simulink model "nnROSNode"  (R2019a)
settings: Solver=FixedStepAuto  StartTime=0.0  StopTime=inf  FixedStep=0.1667  RelTol=1e-3
model workspace (MAT data in the model file):
  SL_ROS_VariableLengthArrays_MaxSizes.CommonInfo.ArrayTruncateAction = 'EmitWarning'
  SL_ROS_VariableLengthArrays_MaxSizes.MsgTypeMap = containers.Map
  SL_ROS_VariableLengthArrays_MaxSizes.MsgTypeMap.serialization.keys = {'dronecomms/droneOut32', 'dronecomms/pidIn32', 'rospy_tutorials/Floats', 'std_msgs/Float32MultiArray'}
  SL_ROS_VariableLengthArrays_MaxSizes.MsgTypeMap.serialization.values{1}.PropertyName = 'Data'
  SL_ROS_VariableLengthArrays_MaxSizes.MsgTypeMap.serialization.values{1}.DataType = 'single'
  SL_ROS_VariableLengthArrays_MaxSizes.MsgTypeMap.serialization.values{1}.MaxLength = 20
  SL_ROS_VariableLengthArrays_MaxSizes.MsgTypeMap.serialization.values{2}.PropertyName = 'Data'
  SL_ROS_VariableLengthArrays_MaxSizes.MsgTypeMap.serialization.values{2}.DataType = 'single'
  SL_ROS_VariableLengthArrays_MaxSizes.MsgTypeMap.serialization.values{2}.MaxLength = 16
  SL_ROS_VariableLengthArrays_MaxSizes.MsgTypeMap.serialization.values{3}.PropertyName = 'Data'
  SL_ROS_VariableLengthArrays_MaxSizes.MsgTypeMap.serialization.values{3}.DataType = 'single'
  SL_ROS_VariableLengthArrays_MaxSizes.MsgTypeMap.serialization.values{3}.MaxLength = 20
  SL_ROS_VariableLengthArrays_MaxSizes.MsgTypeMap.serialization.values{4}.PropertyName = 'Data'
  SL_ROS_VariableLengthArrays_MaxSizes.MsgTypeMap.serialization.values{4}.DataType = 'single'
  SL_ROS_VariableLengthArrays_MaxSizes.MsgTypeMap.serialization.values{4}.MaxLength = 16
  SL_ROS_VariableLengthArrays_MaxSizes.MsgTypeMap.serialization.uniformity = 0
  SL_ROS_VariableLengthArrays_MaxSizes.MsgTypeMap.serialization.keyType = 'char'
  SL_ROS_VariableLengthArrays_MaxSizes.MsgTypeMap.serialization.valueType = 'any'
values from neighbouring files (symbols this model uses):
  maxDeviationTarget = [0.1 0.1 0.1]    [oldNN.mat]
undefined symbols (not defined in the file or in its folder): Data, Data_SL_Info, g, rho, Vehicle
libraries: neural x70, robotlib x3, dspstat3 x2, dynamicsLibrary x1, sharedtransform x1
(part 1 of 2)

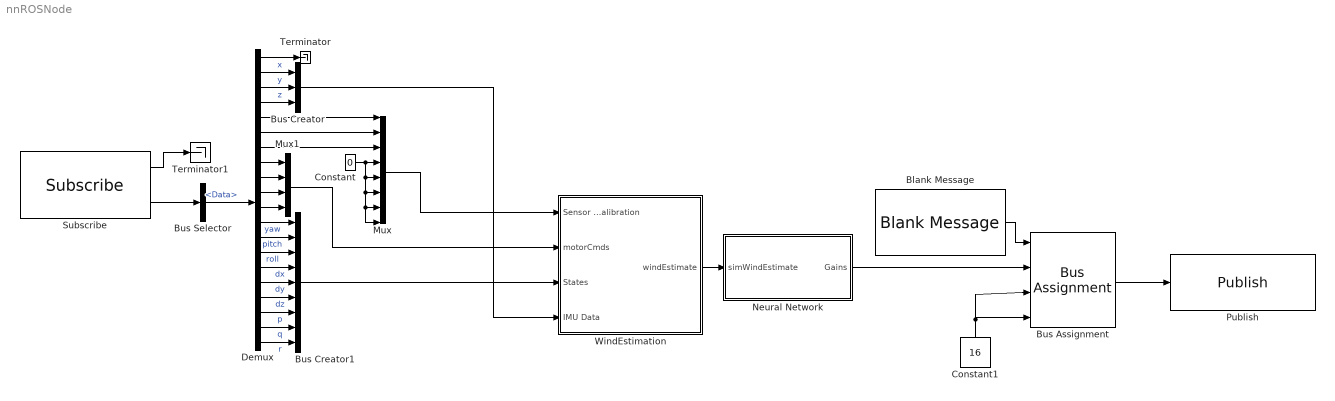
== system nnROSNode ==
  Blank Message : robotlib/Blank Message  messageClass=Message  entityType=dronecomms/pidIn32  messageType=dronecomms/pidIn32  SampleTime=inf
  Bus Assignment : BusAssignment  AssignedSignals=Data,Data_SL_Info.CurrentLength,Data_SL_Info.ReceivedLength
  Bus Creator : BusCreator  Inputs=3
  Bus Creator1 : BusCreator  Inputs=9
  Bus Selector : BusSelector  OutputSignals=Data
  Constant : Constant  Value=0  OutDataTypeStr=single
  Constant1 : Constant  Value=16  OutDataTypeStr=uint32
  Demux : Demux  Outputs=20
  Mux : Mux  Inputs=8
  Mux1 : Mux
  Neural Network : Subsystem
  Publish : robotlib/Publish  topicSource=Specify your own  topic=/pid_gains  messageType=dronecomms/pidIn32  messageQueueLength=1
  Subscribe : robotlib/Subscribe  topicSource=Select from ROS network  topic=/drone_data_recieved  messageType=dronecomms/droneOut32  sampleTime=-1  messageQueueLength=1
  Terminator : Terminator
  Terminator1 : Terminator
  WindEstimation : Subsystem
  wires:
  WindEstimation/1(windEstimate) -> Neural Network/1(simWindEstimate)
  Demux/2 -> Bus Creator/1  "x"
  Demux/3 -> Bus Creator/2  "y"
  Demux/4 -> Bus Creator/3  "z"
  Demux/1 -> Terminator/1
  Demux/8 -> Mux1/1
  Demux/9 -> Mux1/2
  Demux/10 -> Mux1/3
  Demux/11 -> Mux1/4
  Demux/12 -> Bus Creator1/1  "yaw"
  Demux/13 -> Bus Creator1/2  "pitch"
  Demux/14 -> Bus Creator1/3  "roll"
  Demux/15 -> Bus Creator1/4  "dx"
  Demux/16 -> Bus Creator1/5  "dy"
  Demux/17 -> Bus Creator1/6  "dz"
  Demux/18 -> Bus Creator1/7  "p"
  Demux/19 -> Bus Creator1/8  "q"
  Demux/20 -> Bus Creator1/9  "r"
  Demux/5 -> Mux/1
  Demux/6 -> Mux/2
  Demux/7 -> Mux/3
  Mux/1 -> WindEstimation/1(Sensor Calibration)
  Constant/1 -> Mux/8, Mux/7, Mux/6, Mux/5, Mux/4
  Mux1/1 -> WindEstimation/2(motorCmds)
  Bus Creator1/1 -> WindEstimation/3(States)
  Bus Creator/1 -> WindEstimation/4(IMU Data)
  Blank Message/1 -> Bus Assignment/1
  Bus Assignment/1 -> Publish/1
  Neural Network/1(Gains) -> Bus Assignment/2
  Subscribe/1 -> Terminator1/1
  Bus Selector/1 -> Demux/1  "<Data>"
  Constant1/1 -> Bus Assignment/4, Bus Assignment/3
  Subscribe/2 -> Bus Selector/1

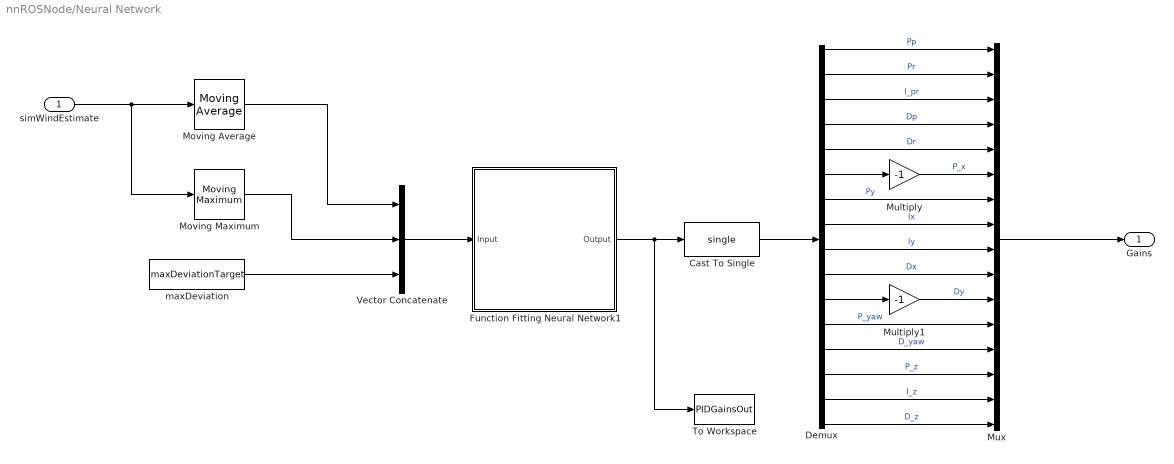
== system nnROSNode/Neural Network ==
  simWindEstimate : Inport
  Cast To Single : DataTypeConversion  OutDataTypeStr=single
  Demux : Demux  Outputs=16
  Function Fitting Neural Network1 : Subsystem
      mask help: Function Fitting Neural Network
  Moving Average : dspstat3/Moving Average  Method=Sliding window  ForgettingFactorPort=off  SpecifyWindowLength=on  WindowLength=100  ForgettingFactor=0.9  SimulateUsing=Code generation
  Moving Maximum : dspstat3/Moving Maximum  SpecifyWindowLength=on  WindowLength=100  SimulateUsing=Code generation
  Multiply : Gain  Gain=-1
  Multiply1 : Gain  Gain=-1
  Mux : Mux  Inputs=16
  To Workspace : ToWorkspace  VariableName=PIDGainsOut  SaveFormat=Structure With Time  SampleTime=-1
  Vector Concatenate : Concatenate  NumInputs=3
  maxDeviation : Constant  Value=maxDeviationTarget
  Gains : Outport
  wires:
  Demux/11 -> Multiply1/1
  Demux/6 -> Multiply/1
  Moving Average/1 -> Vector Concatenate/1
  simWindEstimate/1 -> Moving Maximum/1, Moving Average/1
  maxDeviation/1 -> Vector Concatenate/3
  Function Fitting Neural Network1/1(Output) -> To Workspace/1, Cast To Single/1
  Moving Maximum/1 -> Vector Concatenate/2
  Cast To Single/1 -> Demux/1
  Demux/1 -> Mux/1  "Pp"
  Demux/2 -> Mux/2  "Pr"
  Demux/3 -> Mux/3  "I_pr"
  Demux/4 -> Mux/4  "Dp"
  Demux/5 -> Mux/5  "Dr"
  Multiply/1 -> Mux/6  "P_x"
  Multiply1/1 -> Mux/11  "Dy"
  Demux/7 -> Mux/7  "Py"
  Demux/8 -> Mux/8  "Ix"
  Demux/9 -> Mux/9  "Iy"
  Demux/10 -> Mux/10  "Dx"
  Demux/12 -> Mux/12  "P_yaw"
  Demux/13 -> Mux/13  "D_yaw"
  Demux/14 -> Mux/14  "P_z"
  Demux/15 -> Mux/15  "I_z"
  Demux/16 -> Mux/16  "D_z"
  Vector Concatenate/1 -> Function Fitting Neural Network1/1(Input)
  Mux/1 -> Gains/1

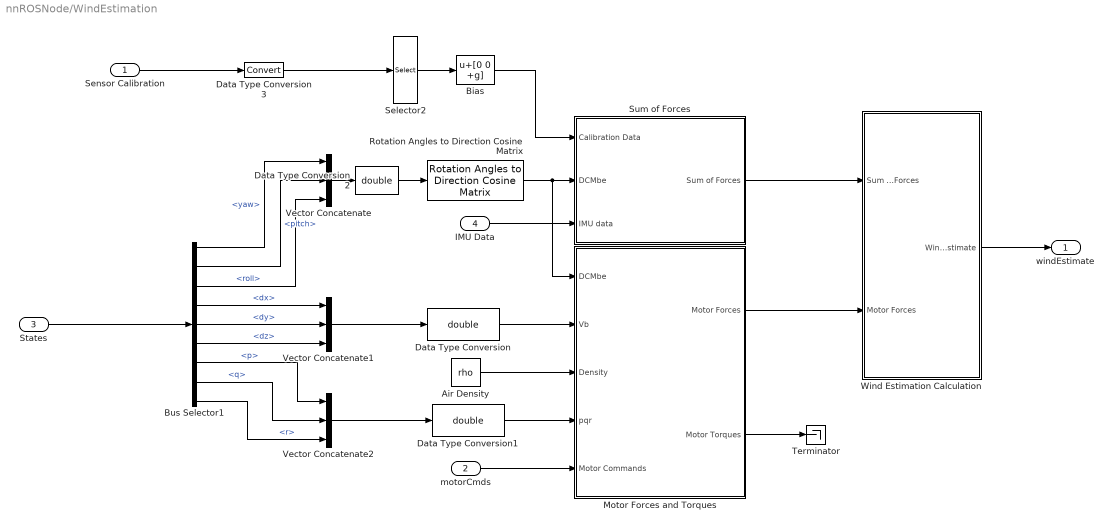
== system nnROSNode/WindEstimation ==
  Sensor Calibration : Inport
  motorCmds : Inport  Port=2
  States : Inport  Port=3
  IMU Data : Inport  Port=4
  Air Density : Constant  Value=rho
  Bias : Bias  Bias=[0 0 +g]
  Bus Selector1 : BusSelector  OutputSignals=yaw,pitch,roll,dx,dy,dz,p,q,r
  Data Type Conversion : DataTypeConversion  OutDataTypeStr=double
  Data Type Conversion1 : DataTypeConversion  OutDataTypeStr=double
  Data Type Conversion2 : DataTypeConversion  OutDataTypeStr=double
  Data Type Conversion3 : DataTypeConversion
  Motor Forces and Torques : Subsystem
  Rotation Angles to Direction Cosine Matrix : sharedtransform/Rotation Angles to Direction Cosine Matrix  rotationOrder=ZYX  aMode=aMode
  Selector2 : Selector  InputPortWidth=8  IndexOptions=Index vector (dialog)  Indices=[1:3]  OutputSizes=1
  Sum of Forces : Subsystem
  Terminator : Terminator
  Vector Concatenate : Concatenate  NumInputs=3
  Vector Concatenate1 : Concatenate  NumInputs=3
  Vector Concatenate2 : Concatenate  NumInputs=3
  Wind Estimation Calculation : Subsystem
  windEstimate : Outport
  wires:
  Sum of Forces/1(Sum of Forces) -> Wind Estimation Calculation/1(Sum of Forces)
  Motor Forces and Torques/1(Motor Forces) -> Wind Estimation Calculation/2(Motor Forces)
  Air Density/1 -> Motor Forces and Torques/3(Density)
  Vector Concatenate/1 -> Data Type Conversion2/1
  Rotation Angles to Direction Cosine Matrix/1 -> Sum of Forces/2(DCMbe), Motor Forces and Torques/1(DCMbe)
  Bus Selector1/4 -> Vector Concatenate1/1  "<dx>"
  Bus Selector1/5 -> Vector Concatenate1/2  "<dy>"
  Bus Selector1/6 -> Vector Concatenate1/3  "<dz>"
  Vector Concatenate1/1 -> Data Type Conversion/1
  Bus Selector1/7 -> Vector Concatenate2/1  "<p>"
  Bus Selector1/8 -> Vector Concatenate2/2  "<q>"
  Bus Selector1/9 -> Vector Concatenate2/3  "<r>"
  Vector Concatenate2/1 -> Data Type Conversion1/1
  Wind Estimation Calculation/1(Wind Estimate) -> windEstimate/1
  IMU Data/1 -> Sum of Forces/3(IMU data)
  motorCmds/1 -> Motor Forces and Torques/5(Motor Commands)
  Motor Forces and Torques/2(Motor Torques) -> Terminator/1
  Data Type Conversion/1 -> Motor Forces and Torques/2(Vb)
  Data Type Conversion1/1 -> Motor Forces and Torques/4(pqr)
  Data Type Conversion2/1 -> Rotation Angles to Direction Cosine Matrix/1
  Bus Selector1/1 -> Vector Concatenate/1  "<yaw>"
  Bus Selector1/2 -> Vector Concatenate/2  "<pitch>"
  Bus Selector1/3 -> Vector Concatenate/3  "<roll>"
  Sensor Calibration/1 -> Data Type Conversion3/1
  Data Type Conversion3/1 -> Selector2/1
  States/1 -> Bus Selector1/1
  Selector2/1 -> Bias/1
  Bias/1 -> Sum of Forces/1(Calibration Data)

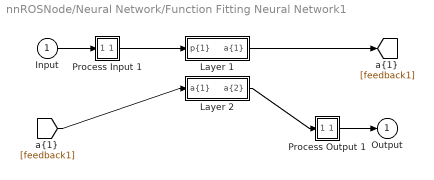
== system nnROSNode/Neural Network/Function Fitting Neural Network1 ==
  Input : Inport  PortDimensions=9
  Layer 1 : Subsystem
  Layer 2 : Subsystem
  Process Input 1 : Subsystem
  Process Output 1 : Subsystem
  Output : Outport  InitialOutput=[0;0;0;0;0;0;0;0;0;0;0;0;0;0;0;0]
  wires:
  Input/1 -> Process Input 1/1(x)
  Process Output 1/1(y) -> Output/1
  Process Input 1/1(p) -> Layer 1/1("p{1}")
  Layer 1/1("a{1}") -> [feedback1]
  [feedback1] -> Layer 2/1("a{1} ")
  Layer 2/1("a{2}") -> Process Output 1/1(a)

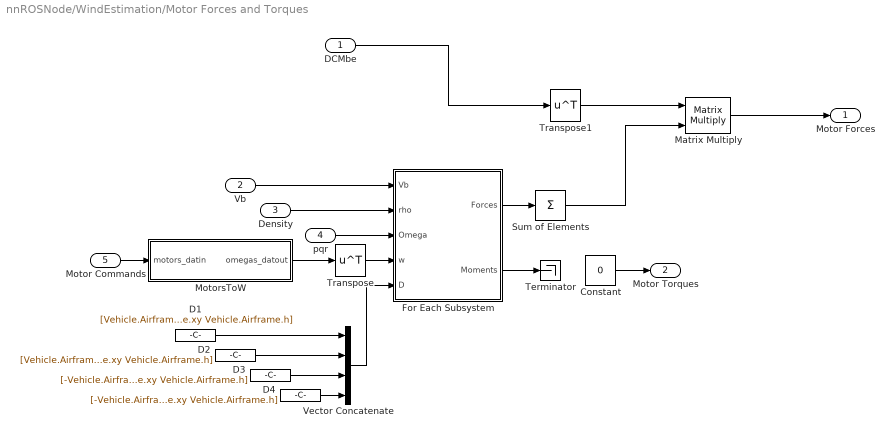
== system nnROSNode/WindEstimation/Motor Forces and Torques ==
  DCMbe : Inport
  Vb : Inport  Port=2
  Density : Inport  Port=3
  pqr : Inport  Port=4
  Motor Commands : Inport  Port=5
  Constant : Constant  Value=0
  D1 : Constant  Value=[Vehicle.Airframe.xy -Vehicle.Airframe.xy Vehicle.Airframe.h]
  D2 : Constant  Value=[Vehicle.Airframe.xy Vehicle.Airframe.xy Vehicle.Airframe.h]
  D3 : Constant  Value=[-Vehicle.Airframe.xy Vehicle.Airframe.xy Vehicle.Airframe.h]
  D4 : Constant  Value=[-Vehicle.Airframe.xy -Vehicle.Airframe.xy Vehicle.Airframe.h]
  For Each Subsystem : Subsystem  TreatAsAtomicUnit=on
  Matrix Multiply : Product  Multiplication=Matrix(*)
  MotorsToW : Subsystem
  Sum of Elements : Sum  Inputs=+  CollapseMode=Specified dimension  CollapseDim=2
  Terminator : Terminator
  Transpose : Math  Operator=transpose  SaturateOnIntegerOverflow=on
  Transpose1 : Math  Operator=transpose  SaturateOnIntegerOverflow=on
  Vector Concatenate : Concatenate  NumInputs=4  Mode=Multidimensional array  ConcatenateDimension=2
  Motor Forces : Outport  Unit=N
  Motor Torques : Outport  Port=2  Unit=N*m
  wires:
  D4/1 -> Vector Concatenate/4
  MotorsToW/1(omegas_datout) -> Transpose/1
  Vector Concatenate/1 -> For Each Subsystem/5(D)
  For Each Subsystem/2(Moments) -> Terminator/1
  pqr/1 -> For Each Subsystem/3(Omega)
  Vb/1 -> For Each Subsystem/1(Vb)
  Motor Commands/1 -> MotorsToW/1(motors_datin)
  D1/1 -> Vector Concatenate/1
  D3/1 -> Vector Concatenate/3
  D2/1 -> Vector Concatenate/2
  Density/1 -> For Each Subsystem/2(rho)
  For Each Subsystem/1(Forces) -> Sum of Elements/1
  Transpose/1 -> For Each Subsystem/4(w)
  DCMbe/1 -> Transpose1/1
  Sum of Elements/1 -> Matrix Multiply/2
  Matrix Multiply/1 -> Motor Forces/1
  Constant/1 -> Motor Torques/1
  Transpose1/1 -> Matrix Multiply/1

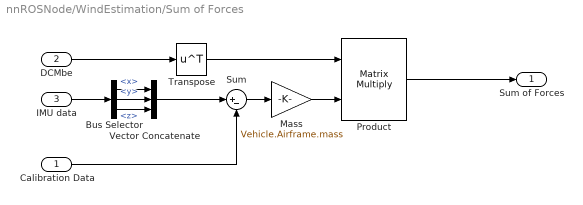
== system nnROSNode/WindEstimation/Sum of Forces ==
  Calibration Data : Inport
  DCMbe : Inport  Port=2
  IMU data : Inport  Port=3
  Bus Selector : BusSelector  OutputSignals=x,y,z
  Mass : Gain  Gain=Vehicle.Airframe.mass
  Product : Product  Multiplication=Matrix(*)
  Sum : Sum  Inputs=|+-
  Transpose : Math  Operator=transpose  SaturateOnIntegerOverflow=on
  Vector Concatenate : Concatenate  NumInputs=3
  Sum of Forces : Outport
  wires:
  Mass/1 -> Product/2
  Product/1 -> Sum of Forces/1
  DCMbe/1 -> Transpose/1
  Transpose/1 -> Product/1
  Sum/1 -> Mass/1
  Calibration Data/1 -> Sum/2
  IMU data/1 -> Bus Selector/1
  Bus Selector/1 -> Vector Concatenate/1  "<x>"
  Bus Selector/2 -> Vector Concatenate/2  "<y>"
  Bus Selector/3 -> Vector Concatenate/3  "<z>"
  Vector Concatenate/1 -> Sum/1

== system nnROSNode/WindEstimation/Wind Estimation Calculation ==
  Sum of Forces : Inport  Unit=N
  Motor Forces : Inport  Port=2  Unit=N
  Add1 : Sum  Inputs=-+
  Signal Specification : SignalSpecification  Dimensions=3
  Wind Estimate : Outport  Unit=N
  wires:
  Add1/1 -> Signal Specification/1
  Motor Forces/1 -> Add1/2  "Motor Thrust"
  Signal Specification/1 -> Wind Estimate/1
  Sum of Forces/1 -> Add1/1

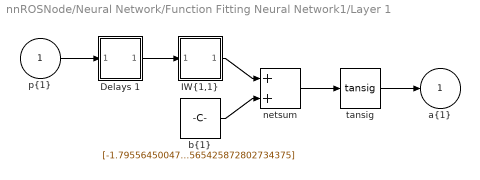
== system nnROSNode/Neural Network/Function Fitting Neural Network1/Layer 1 ==
  "p{1}" : Inport  PortDimensions=9
  Delays 1 : Subsystem
  "IW{1,1}" : Subsystem
  "b{1}" : Constant  Value=[-1.7955645004714162471515237484709359705448150634765625;-2.15497494357021412980657260050065815448760986328125;-5.1640507279492577907831218908540904521942138671875;-2.76294672593349144307239839690737426280975341796875;-3.97972555528513627365327920415438711643218994140625;1.5357575601541004761685371704516001045703887939453125;-2.41842359798930051084653314319439232349395751953125;-3.069728140043751718479825285612605512142181396484375;2.3434017526420927168828711728565394878387451171875;-3.33356323179282387769717388437129557132720947265625;-2.298045377366748187597522701253183186054229736328125;-1.0429336870214711563420451057027094066143035888671875;-2.547726845174876242339223608723841607570648193359375;1.697470253943376139460497142863459885120391845703125;-0.49817549652620407574232785918866284191608428955078125;0.2086056696170743018914350841441773809492588043212890625;1.4087452224027761094049537859973497688770294189453125;0.581284941699784507562753788079135119915008544921875;-0.8166567672995450610784473610692657530307769775390625;-0.728099088247456283085057293646968901157379150390625;-3.4228858918562448110378682031296193599700927734375;-0.54450534677862261201397586773964576423168182373046875;1.8563456105631608306083535353536717593669891357421875;0.6346380653648571179559212396270595490932464599609375;0.259453839281130804739206041631405241787433624267578125;2.01189893107739958821866821381263434886932373046875;0.56436382436911569637771890484145842492580413818359375;0.281991500226897784386892453767359256744384765625;-0.65570427209520365519068718640482984483242034912109375;0.3550983989298384102539785089902579784393310546875;-3.889413959690978028760355300619266927242279052734375;2.817466039075230188615250881412066519260406494140625;-1.1468025296414092739638590501272119581699371337890625;1.7379312480090367554197428034967742860317230224609375;-1.579820375847007962732959640561603009700775146484375;1.2380323493480964724966497669811360538005828857421875;0.59337685282001662034900846265372820198535919189453125;1.0788776954776977401451176774571649730205535888671875;-1.3404241065343802663534233943209983408451080322265625;-1.3597799544942585914242272338015027344226837158203125;1.91486334262139212825104550574906170368194580078125;2.088984064741117752106447369442321360111236572265625;-1.839289848699215301763842944637872278690338134765625;1.541336103742971364027880554203875362873077392578125;1.158088050538635283004396114847622811794281005859375;-1.936653531678591999565242076641879975795745849609375;5.67596610769249565464633633382618427276611328125;-2.2834014697268241178562675486318767070770263671875;-2.457924527770686484728912546415813267230987548828125;-4.08661248344289873557499959133565425872802734375]
  netsum : Sum  Inputs=2  SaturateOnIntegerOverflow=on  InputSameDT=on  OutDataTypeStr=Inherit: Same as first input
  tansig : neural/Transfer Functions/tansig
  "a{1}" : Outport  InitialOutput=[0;0;0;0;0;0;0;0;0;0;0;0;0;0;0;0;0;0;0;0;0;0;0;0;0;0;0;0;0;0;0;0;0;0;0;0;0;0;0;0;0;0;0;0;0;0;0;0;0;0]
  wires:
  "p{1}"/1 -> Delays 1/1("p{1}")
  Delays 1/1("pd{1,1}") -> "IW{1,1}"/1("pd{1,1}")
  "IW{1,1}"/1("iz{1,1}") -> netsum/1
  "b{1}"/1 -> netsum/2
  netsum/1 -> tansig/1
  tansig/1 -> "a{1}"/1

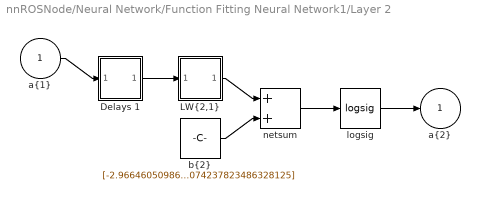
== system nnROSNode/Neural Network/Function Fitting Neural Network1/Layer 2 ==
  "a{1} " : Inport  PortDimensions=50
  Delays 1 : Subsystem
  "LW{2,1}" : Subsystem
  "b{2}" : Constant  Value=[-2.966460509866037487114454052061773836612701416015625;2.207572265518088716618194666807539761066436767578125;-2.278026460671383812695012238691560924053192138671875;-1.7701088589645299631314401267445646226406097412109375;1.3396075502919984057115243558655492961406707763671875;0.324384695762535313345864551592967472970485687255859375;0.0229326543932350211674187079324838123284280300140380859375;-0.11018893637483805070242937063085264526307582855224609375;-0.1844907086015066532969086665616487152874469757080078125;0.28179023726584373488179835476330481469631195068359375;-1.4775688630826497860226709235575981438159942626953125;1.2963054540746059561939773630001582205295562744140625;-1.7830992323228669338419649648130871355533599853515625;1.2133783210993163148572193676955066621303558349609375;-3.053949478411235762820297168218530714511871337890625;-3.7697587775003729149148057331331074237823486328125]
  logsig : neural/Transfer Functions/logsig
  netsum : Sum  Inputs=2  SaturateOnIntegerOverflow=on  InputSameDT=on  OutDataTypeStr=Inherit: Same as first input
  "a{2}" : Outport  InitialOutput=[0;0;0;0;0;0;0;0;0;0;0;0;0;0;0;0]
  wires:
  "a{1} "/1 -> Delays 1/1("p{2}")
  Delays 1/1("pd{2,1}") -> "LW{2,1}"/1("ad{2,1}")
  "LW{2,1}"/1("lz{2,1}") -> netsum/1
  "b{2}"/1 -> netsum/2
  netsum/1 -> logsig/1
  logsig/1 -> "a{2}"/1

== system nnROSNode/Neural Network/Function Fitting Neural Network1/Process Input 1 ==
  x : Inport  PortDimensions=9
  mapminmax : neural/Processing Functions/mapminmax  xmin=[-0.144320129611064745800419473198;-0.146407166837474983500655412172;-0.030419447754752425988611364005;0.0566263432042784509157229422271;0.0545760904858537398975926180356;0.0614873201862948803864128421992;0.00621446561439853439878788776696;0.00386812285744042583246482536197;0.0400257857899877222962459200062]  xmax=[0.151629203383399635551853634752;0.147424314816403473349382124979;0.00285287611269392088475527202718;0.884807520475853870323135197395;0.640221310211877225881949016184;0.378940784357309490282261776883;9.20630362144751046571400365792;8.46022302243510182506724959239;1.19241761272227786427890805498]  ymin=-1  ymax=1
  p : Outport  PortDimensions=9
  wires:
  x/1 -> mapminmax/1
  mapminmax/1 -> p/1

== system nnROSNode/Neural Network/Function Fitting Neural Network1/Process Output 1 ==
  a : Inport  PortDimensions=16
  mapminmax_reverse : neural/Processing Functions/mapminmax_reverse  xmin=[0.000351411811559587639822860305472;0.000351411811559587639822860305472;2.66503509516180535713887698318e-07;2.0987980606623769362147774193e-07;2.0987980606623769362147774193e-07;2.82978912491405054652204853483e-05;2.82978912491405054652204853483e-05;7.16898254142783758767519877719e-06;7.16898254142783758767519877719e-06;0.00113586863338273054251092997191;0.00113586863338273054251092997191;5.14555055560750348123556351804e-07;5.85310891857426803448172475224e-08;0.000240423520823762615350460691843;3.82866893686717446598777314648e-05;0.000264068851819510008738234319026]  xmax=[0.0299990456964187510169317363307;0.0299990456964187510169317363307;0.019995974274727417591135392172;0.00499872503694963245951532471167;0.00499872503694963245951532471167;0.499682080443875187292235295899;0.499682080443875187292235295899;0.0999985933870808363366222693003;0.0999985933870808363366222693003;0.299913637646852637708150268736;0.299913637646852637708150268736;0.00999633631343448125772255252741;0.0029998731430596740389626919665;1.99986952250969696187610225024;0.999990563439456137118099832151;0.999960970515257230317729408853]  ymin=-1  ymax=1
  y : Outport  PortDimensions=16
  wires:
  a/1 -> mapminmax_reverse/1
  mapminmax_reverse/1 -> y/1

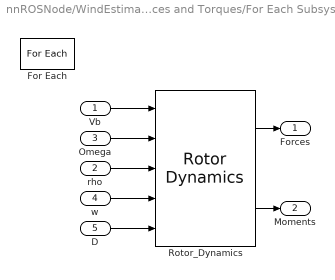
== system nnROSNode/WindEstimation/Motor Forces and Torques/For Each Subsystem ==
  Vb : Inport  PortDimensions=3
  rho : Inport  Port=2  PortDimensions=1
  Omega : Inport  Port=3
  w : Inport  Port=4  Partition=on  PartitionDimension=2  PartitionWidth=1  PartitionOffset=0
  D : Inport  Port=5  Partition=on  PartitionDimension=2  PartitionWidth=1  PartitionOffset=0
  For Each : ForEach  DisableCoverage=on  IndexMode=One-based
  Rotor_Dynamics : dynamicsLibrary/Rotor Dynamics  SystemSampleTime=-1
  Forces : Outport  ConcatenationDimension=2
  Moments : Outport  Port=2  ConcatenationDimension=2
  wires:
  Rotor_Dynamics/1 -> Forces/1
  Rotor_Dynamics/2 -> Moments/1
  Vb/1 -> Rotor_Dynamics/1
  Omega/1 -> Rotor_Dynamics/2
  rho/1 -> Rotor_Dynamics/3
  D/1 -> Rotor_Dynamics/5
  w/1 -> Rotor_Dynamics/4

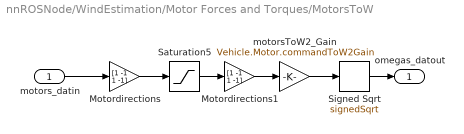
== system nnROSNode/WindEstimation/Motor Forces and Torques/MotorsToW ==
  motors_datin : Inport
  Motordirections : Gain  Gain=[1 -1 1 -1]  ParamDataTypeStr=single  OutDataTypeStr=Inherit: Inherit via back propagation  SaturateOnIntegerOverflow=on
  Motordirections1 : Gain  Gain=[1 -1 1 -1]  ParamDataTypeStr=single  OutDataTypeStr=Inherit: Inherit via back propagation  SaturateOnIntegerOverflow=on
  Saturation5 : Saturate  UpperLimit=Vehicle.Motor.maxLimit  LowerLimit=Vehicle.Motor.minLimit  OutDataTypeStr=Inherit: Inherit via back propagation
  Signed Sqrt : Sqrt  Operator=signedSqrt  OutDataTypeStr=Inherit: Inherit via back propagation  SaturateOnIntegerOverflow=on
  motorsToW2_Gain : Gain  Gain=Vehicle.Motor.commandToW2Gain  ParamDataTypeStr=single  OutDataTypeStr=Inherit: Inherit via back propagation  SaturateOnIntegerOverflow=on
  omegas_datout : Outport
  wires:
  motorsToW2_Gain/1 -> Signed Sqrt/1
  Motordirections/1 -> Saturation5/1
  Saturation5/1 -> Motordirections1/1
  Motordirections1/1 -> motorsToW2_Gain/1
  Signed Sqrt/1 -> omegas_datout/1
  motors_datin/1 -> Motordirections/1

== system nnROSNode/Neural Network/Function Fitting Neural Network1/Layer 1/Delays 1 ==
  "p{1}" : Inport  PortDimensions=9
  mux : Mux  Inputs=1
  "pd{1,1}" : Outport
  wires:
  "p{1}"/1 -> mux/1
  mux/1 -> "pd{1,1}"/1

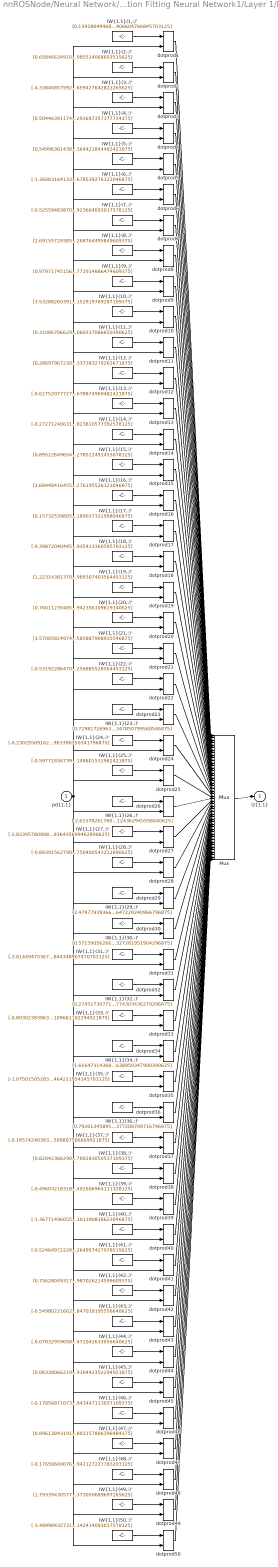
== system nnROSNode/Neural Network/Function Fitting Neural Network1/Layer 1/IW{1,1} ==
  "pd{1,1}" : Inport  PortDimensions=9
  "IW{1,1}(1,:)'" : Constant  Value=[0.1392804946893048956280125594275887124240398406982421875;-4.40865246500433460852264033746905624866485595703125;0.6283017301369773210950597785995341837406158447265625;-0.61074222910749098591765005039633251726627349853515625;2.5562093146691626799338337150402367115020751953125;-0.990206292142548960555359371937811374664306640625;-0.999379572475788346963554431567899882793426513671875;0.35948009547073400682393184979446232318878173828125;-0.1235236564405906012353852929663844406604766845703125]
  "IW{1,1}(10,:)'" : Constant  Value=[3.53288260391285202643985030590556561946868896484375;0.499543784873980711846996882741223089396953582763671875;1.0323925645887708224535117551567964255809783935546875;0.88578370351871515975261672792839817702770233154296875;2.236130373036990359736364553100429475307464599609375;0.034781493053705973828026998262430424802005290985107421875;-3.59937276079998103028856348828412592411041259765625;3.167800444255937986071103296126239001750946044921875;-5.7497523294883734479299164377152919769287109375]
  "IW{1,1}(11,:)'" : Constant  Value=[0.3108670662966976916408157194382511079311370849609375;0.171379936987389014380056551090092398226261138916015625;0.6010662407850648758511624691891483962535858154296875;1.277863444962637817781114790705032646656036376953125;-1.16664262014854447357947719865478575229644775390625;0.2739598565265228824472387714195065200328826904296875;0.135289766018030499505897523704334162175655364990234375;-2.96675359846638375671545873046852648258209228515625;-0.15101352485950025883454372888081707060337066650390625]
  "IW{1,1}(12,:)'" : Constant  Value=[0.28697967230990417686342652814346365630626678466796875;0.87488597850220262142073579525458626449108123779296875;1.3815512432980459056608424361911602318286895751953125;0.01602359542899843558583228286806843243539333343505859375;-1.066579399432118435697702807374298572540283203125;0.60115746312273110607549142514471895992755889892578125;3.316271516247191630810675633256323635578155517578125;-2.0682964937997194709851100924424827098846435546875;0.4696813139281743598729690347681753337383270263671875]
  "IW{1,1}(13,:)'" : Constant  Value=[-0.62752077727405464191434703025151975452899932861328125;0.29778697648318530610822563176043331623077392578125;0.21902019338279588023254973450093530118465423583984375;1.0459585999213973916965869648265652358531951904296875;1.025635406552062089957644275273196399211883544921875;-2.43582477820745690877402012120001018047332763671875;-2.6572711724044353331919410265982151031494140625;-0.431472478972530881780045319828786887228488922119140625;1.91301219425728685763488101656548678874969482421875]
  "IW{1,1}(14,:)'" : Constant  Value=[-0.272712406312350774673092246302985586225986480712890625;0.01524796993062578660815820086327221360988914966583251953125;-1.5558772094552308917769778418005444109439849853515625;0.80490879821129712734517624994623474776744842529296875;2.083790136469963361065538265393115580081939697265625;-1.8891608109119442104884001309983432292938232421875;-0.12586322367984548176167436395189724862575531005859375;1.172083262123337465965278170187957584857940673828125;0.10389971286616513090894642346029286272823810577392578125]
  "IW{1,1}(15,:)'" : Constant  Value=[0.895226496547965933103796487557701766490936279296875;1.374769152305139296998959252960048615932464599609375;-0.823325349434176789742423352436162531375885009765625;-1.1817334460802324525019457723828963935375213623046875;0.6655165283322721503367347395396791398525238037109375;0.9782529329588509625637016142718493938446044921875;-1.440155551647622100830403724103234708309173583984375;0.5869894186405935077033291236148215830326080322265625;1.675826502866577971673223146353848278522491455078125]
  "IW{1,1}(16,:)'" : Constant  Value=[2.684484164558389007737559950328432023525238037109375;-1.7457054346212059758869372672052122652530670166015625;1.588693262955388707524662095238454639911651611328125;-2.236440082675930529632069010403938591480255126953125;-1.694753134166165242646684419014491140842437744140625;0.31357419736420844014190834059263579547405242919921875;3.22809278077587169519802046124823391437530517578125;-2.580450087459348562646255231811664998531341552734375;3.582728997579859520072886880370788276195526123046875]
  "IW{1,1}(17,:)'" : Constant  Value=[0.1573253980557753617386396172150853089988231658935546875;1.9568180619977173506640610867179930210113525390625;0.0428616364074436984044069731680792756378650665283203125;0.76370576971549386513515855767764151096343994140625;1.4300284217267940078954779892228543758392333984375;1.095693350470374749505708678043447434902191162109375;-0.12117535270433606175988217046324280090630054473876953125;-0.65341761371514961442841240568668581545352935791015625;0.42403507126661021953140107143553905189037322998046875]
  "IW{1,1}(18,:)'" : Constant  Value=[-0.398720404451288867875291543896310031414031982421875;0.64395394117870019545790682968799956142902374267578125;-0.472134122560477320629246378302923403680324554443359375;-0.23305116054581731521722076649894006550312042236328125;-0.2307066364255479784528546360888867639005184173583984375;-0.9832988984260462306252748021506704390048980712890625;-0.9721304472999445778214067104272544384002685546875;-0.550182395676989788313449025736190378665924072265625;-1.234963383617543541959094000048935413360595703125]
  "IW{1,1}(19,:)'" : Constant  Value=[1.223143813707142424362928068148903548717498779296875;-1.3174998317158863603282270560157485306262969970703125;-1.3126758872151926826887802235432900488376617431640625;-0.398150324534760235994923505131737329065799713134765625;1.34442024544624683102256312849931418895721435546875;0.1082381421897620210614832103601656854152679443359375;-1.2978159627494936234626266013947315514087677001953125;-1.228074070035687359592202483327127993106842041015625;-0.140743026658573189280332371708936989307403564453125]
  "IW{1,1}(2,:)'" : Constant  Value=[0.65846634910639656457220780794159509241580963134765625;0.71444337130805857238868838976486586034297943115234375;-0.5211983936811035444947037831298075616359710693359375;0.1503415980478204627690530514882993884384632110595703125;0.446361314458301572383192024062736891210079193115234375;-0.311213721908170481977862209532759152352809906005859375;1.082448478785274392777182583813555538654327392578125;0.646158002831836331125714423251338303089141845703125;1.213745191788986321768106790841557085514068603515625]
  "IW{1,1}(20,:)'" : Constant  Value=[0.760112354858593075590533771901391446590423583984375;2.445855792499167957743111401214264333248138427734375;-2.24480414588414500798307926743291318416595458984375;0.46533493781938395361663651783601380884647369384765625;-0.332488874221646357742798727485933341085910797119140625;-1.66159676341970996560348794446326792240142822265625;-1.0016287410436095495214203765499405562877655029296875;0.371492114631901515497958143896539695560932159423828125;-1.34718331479631903135896209278143942356109619140625]
  "IW{1,1}(21,:)'" : Constant  Value=[3.570058249745971412636436070897616446018218994140625;-0.148607961247463504772525766384205780923366546630859375;-1.152856541249821731298652593977749347686767578125;-1.21011463215943404492236368241719901561737060546875;3.53115762703990210269466842873953282833099365234375;5.69766969203461570714353001676499843597412109375;-1.213194549582477410609726575785316526889801025390625;-2.654060890690610907682867036783136427402496337890625;-8.5349603663522639607208475354127585887908935546875]
  "IW{1,1}(22,:)'" : Constant  Value=[-0.5319228647013345412375429077656008303165435791015625;0.64319525422771361977680726340622641146183013916015625;-1.3493919685558382060008852931787259876728057861328125;0.08317909057212613532783507253043353557586669921875;1.357273232990702904743329781922511756420135498046875;0.5576747313158991747883419520803727209568023681640625;0.772015138821135149527208341169171035289764404296875;-0.0694246524193254666013075393493636511266231536865234375;0.70338216293880340135302731141564436256885528564453125]
  "IW{1,1}(23,:)'" : Constant  Value=[0.72981726963356419179973499922198243439197540283203125;-1.7752181296687437050962898865691386163234710693359375;2.715447581628084083860130704124458134174346923828125;1.83682011265025035839926204062066972255706787109375;2.04663018976397115267218396184034645557403564453125;-0.336640523998948448802792654532822780311107635498046875;2.411391079975020890202586087980307638645172119140625;1.96362774592629651948527680360712110996246337890625;-4.9310484735926802812855385127477347850799560546875]
  "IW{1,1}(24,:)'" : Constant  Value=[-0.2302550916252381341120525348742376081645488739013671875;-0.300313428500946166810336990238283760845661163330078125;1.357194592066765626015012458083219826221466064453125;-0.53873769399211635100499506734195165336132049560546875;-0.81913028168569501641371743971831165254116058349609375;-0.464439662475849834866181709003285504877567291259765625;-0.6020674602320774670971559316967613995075225830078125;-0.0757461055274451233731980437369202263653278350830078125;-1.109576663439202359739965686458162963390350341796875]
  "IW{1,1}(25,:)'" : Constant  Value=[-0.59771836739643602331994998166919685900211334228515625;0.497440583700314464810077197398641146719455718994140625;-0.253257780980035540618899858600343577563762664794921875;0.97351482963155266947552490819361992180347442626953125;1.0496695340833088749832313624210655689239501953125;-0.55784183022142130869980292118270881474018096923828125;0.36901019464378193024600705030024982988834381103515625;-1.08337618736520102658005271223373711109161376953125;1.4831836666883411179895801979000680148601531982421875]
  "IW{1,1}(26,:)'" : Constant  Value=[-2.61578261760845531824770660023204982280731201171875;-0.7298851450771757232161007777904160320758819580078125;4.1759575142139322423417979734949767589569091796875;-1.1914197200658893649460878805257380008697509765625;-4.87405265653318320318021505954675376415252685546875;-2.817233961758938587394140995456837117671966552734375;1.6578479435357535987094479423831216990947723388671875;2.69148454504240408624582414631731808185577392578125;8.8273006741561577115362524637021124362945556640625]
  "IW{1,1}(27,:)'" : Constant  Value=[-2.833957809082454648574866951094008982181549072265625;-1.162356594803698239815048509626649320125579833984375;4.76333271710702721435382045456208288669586181640625;-0.28637194923981834637771726193022914230823516845703125;-1.275790081287101696005947815137915313243865966796875;-1.6672411313134858357187795263598673045635223388671875;-2.369072725215612518212537906947545707225799560546875;2.303535656283354438045307688298635184764862060546875;6.49734380742379702411426478647626936435699462890625]
  "IW{1,1}(28,:)'" : Constant  Value=[-0.8939156279064153221014521477627567946910858154296875;-0.6768478575199792235395079842419363558292388916015625;-0.5013198850295543795851926915929652750492095947265625;-1.197109217033426542542429160675965249538421630859375;-0.81621125372872038727933841073536314070224761962890625;-1.155703767237884704854877782054245471954345703125;-0.91241465979714886369578152880421839654445648193359375;0.39308477497093041730380491571850143373012542724609375;-0.6228906502731954564211491742753423750400543212890625]
  "IW{1,1}(29,:)'" : Constant  Value=[2.479779393665582087891152696101926267147064208984375;1.6007692897567604717323774821124970912933349609375;-3.8610695611165137819398296414874494075775146484375;0.00441007555756696596749311112262148526497185230255126953125;-4.472478848246527860510468599386513233184814453125;5.47782430969202049908517437870614230632781982421875;0.80487949164375727217901612675632350146770477294921875;-2.01465603258842929079719397122971713542938232421875;-2.338327422690969381591230558115057647228240966796875]
  "IW{1,1}(3,:)'" : Constant  Value=[-4.33846857592165680017615159158594906330108642578125;-0.027689297208241592240796080659492872655391693115234375;-1.31080244611995855308350655832327902317047119140625;1.3599385201902529640705097335739992558956146240234375;-3.385601152134398716953000985085964202880859375;1.0041110646447359844302127385162748396396636962890625;-1.2616832739890233572310762610868550837039947509765625;-0.84335354582018406954802003383520059287548065185546875;-2.45291421955784105790598914609290659427642822265625]
  "IW{1,1}(30,:)'" : Constant  Value=[0.57159056266594010509152212762273848056793212890625;0.2431509442495662642880205339679378084838390350341796875;-1.1916911054682415294081465617637149989604949951171875;0.3160968088457425384518728606053628027439117431640625;-1.8354330587476954672609963381546549499034881591796875;-0.753604670926417696819044067524373531341552734375;-0.51030869061905537176215830186265520751476287841796875;1.076217865643282589616092081996612250804901123046875;-0.556738851284507063610362820327281951904296875]
  "IW{1,1}(31,:)'" : Constant  Value=[-3.814494753670572446679898348520509898662567138671875;0.1997515379931849854866499072159058414399623870849609375;-1.2859749176561237060667508558253757655620574951171875;1.092910767869965216192440493614412844181060791015625;-2.279980538161039849143207902670837938785552978515625;1.92709765437102920060397082124836742877960205078125;3.088658896010717302971215758589096367359161376953125;0.16951033446983931884943785917130298912525177001953125;-7.9992959292992811271005848539061844348907470703125]
  "IW{1,1}(32,:)'" : Constant  Value=[0.27451730771967064459460061698337085545063018798828125;-0.460449534274060490179891758089070208370685577392578125;-1.5150784768473590791160177104757167398929595947265625;-2.614592353434005644885473884642124176025390625;-0.1373476401529509505206050334891187958419322967529296875;2.192427066861721840496102231554687023162841796875;1.0100487165539953071657919281278736889362335205078125;-2.993663673851678641568696548347361385822296142578125;5.67797115931043361314323192345909774303436279296875]
  "IW{1,1}(33,:)'" : Constant  Value=[-0.80302383063299231924503374102641828358173370361328125;-2.003673527295708023387987850583158433437347412109375;-2.439608549044845364761613382142968475818634033203125;1.0828426455012516438358716186485253274440765380859375;-3.865250899178082288898394835996441543102264404296875;-0.73880145560556942374574873610981740057468414306640625;1.996507708259952718066188026568852365016937255859375;1.74304684364491269121799632557667791843414306640625;-1.94079024234219854605498767341487109661102294921875]
  "IW{1,1}(34,:)'" : Constant  Value=[1.616473143681040891550537708099000155925750732421875;1.1106059621391295433312507157097570598125457763671875;1.491484606280144564749434721306897699832916259765625;3.67934337069951045151583457482047379016876220703125;-1.573063868925085984074030420742928981781005859375;-0.79398305840468685889987909831688739359378814697265625;-1.0674876704220792600352751833270303905010223388671875;-1.8769471159635473522797610712586902081966400146484375;3.71491676193608899581022342317737638950347900390625]
  "IW{1,1}(35,:)'" : Constant  Value=[-1.0750150528311437359008095882018096745014190673828125;-3.2906797962690372827410101308487355709075927734375;0.7571881024255151526602958256262354552745819091796875;-0.93064914479459448504172769389697350561618804931640625;2.47931613949176909983407313120551407337188720703125;-2.044902162944187917759109041071496903896331787109375;1.470972360517020405268340255133807659149169921875;-0.99362974302703743756381982166203670203685760498046875;-2.029379480003850932945397289586253464221954345703125]
  "IW{1,1}(36,:)'" : Constant  Value=[0.79201345895830221888189726087148301303386688232421875;-1.8368247781826465558907557351631112396717071533203125;-1.4363641133490803181160799795179627835750579833984375;-0.020367886979015224768740921490461914800107479095458984375;1.3799355304243519082518787399749271571636199951171875;-0.19070382222722359610855846767663024365901947021484375;1.5006013907653825700805327869602479040622711181640625;1.1500394183564519590134977988782338798046112060546875;-0.635897882798321045783040972310118377208709716796875]
  "IW{1,1}(37,:)'" : Constant  Value=[-0.1857424038382916309242176566840498708188533782958984375;-1.992474793940445021434015870909206569194793701171875;-2.4293535532138630372855914174579083919525146484375;-0.089924753395544676504158587704296223819255828857421875;1.297260843361665916262381870183162391185760498046875;1.321434567345367572244185794261284172534942626953125;-3.107420783071018544063690569601021707057952880859375;-0.824749167971388974507362945587374269962310791015625;0.80150970887389838548386933325673453509807586669921875]
  "IW{1,1}(38,:)'" : Constant  Value=[0.820423662906312411990938926464878022670745849609375;0.204199303971046186578774950248771347105503082275390625;-0.5164584222092585275021292545716278254985809326171875;1.0043619085390507184030184362200088798999786376953125;-1.076583326141922203333933794056065380573272705078125;1.1019308785543813211660335582564584910869598388671875;0.0813595401056233791248217812608345411717891693115234375;-0.5978462433345421711550216059549711644649505615234375;-1.0278611193373412557861001914716325700283050537109375]
  "IW{1,1}(39,:)'" : Constant  Value=[-0.496032183180095065377912533222115598618984222412109375;-0.56401415351328354486071248174994252622127532958984375;-0.693749096175519941454012950998730957508087158203125;-0.069158081432482365613623187527991831302642822265625;-1.37339612185064918747912088292650878429412841796875;0.8612453847541281515276523350621573626995086669921875;0.0215135057333350233899071923815426998771727085113525390625;-0.0820992703116190103429516966571100056171417236328125;1.3205548142783272158595764267374761402606964111328125]
  "IW{1,1}(4,:)'" : Constant  Value=[0.5044639117440798958824643705156631767749786376953125;0.403896161907628725717955830987193621695041656494140625;-2.1396479610108602997797788702882826328277587890625;0.42848981560163823534281846150406636297702789306640625;-1.80908197927644476266095807659439742565155029296875;-0.052303766016394449833715185604887665249407291412353515625;-1.7967104668800824018859429997974075376987457275390625;-3.41069084762861951531931481440551578998565673828125;3.563322428121093565778210177086293697357177734375]
  "IW{1,1}(40,:)'" : Constant  Value=[-1.3677149605532132881080542574636638164520263671875;-1.009392365466453167499594201217405498027801513671875;-1.0988910623259366960979832583689130842685699462890625;-0.1662832330043414741371776699452311731874942779541015625;-0.56247960849427169893743894135695882141590118408203125;0.49282387082433753988652824773453176021575927734375;0.365110305289096659375758235910325311124324798583984375;0.04956660607441844279552611851613619364798069000244140625;0.252583924942342885611168412651750259101390838623046875]
  "IW{1,1}(41,:)'" : Constant  Value=[-0.5246497222836088436537238521850667893886566162109375;-2.96868026028598563925697817467153072357177734375;-0.2411013279004350640111198345039156265556812286376953125;0.94924503971880513919501254349597729742527008056640625;-0.479138487595985818057187088925275020301342010498046875;-0.395762688440590981731048714209464378654956817626953125;1.1984534419764278911912924741045571863651275634765625;-1.9219663798521400277508064391440711915493011474609375;1.3541184313997105537197285229922272264957427978515625]
  "IW{1,1}(42,:)'" : Constant  Value=[0.75628049317772683135530087383813224732875823974609375;0.2229968781697820034981560866071959026157855987548828125;-0.45971511167733203340191039387718774378299713134765625;0.2302920181118086606630868118372745811939239501953125;0.74282882629321156375823420603410340845584869384765625;-0.53723614304901456950602778306347317993640899658203125;-0.36571640965756169183720203363918699324131011962890625;-0.632164453239027590569776293705217540264129638671875;-1.3012645323757856541391220162040553987026214599609375]
  "IW{1,1}(43,:)'" : Constant  Value=[-0.54980221662444772601219256102922372519969940185546875;-1.3493913527064738122618337001767940819263458251953125;-0.10308852906945864535970258657471276819705963134765625;-0.62877065977709900579384338925592601299285888671875;-0.38779552390202098877125536091625690460205078125;0.01824614044487289643559080332124722190201282501220703125;-0.665484643258932972997854449204169213771820068359375;-1.7829460431157266864232724401517771184444427490234375;-1.0964082835101722768200716018327511847019195556640625]
  "IW{1,1}(44,:)'" : Constant  Value=[-0.07832959058975395849611089715835987590253353118896484375;1.1444301995817767192420433275401592254638671875;-1.8496455477711071235802364753908477723598480224609375;-0.82717693996606500572710274354903958737850189208984375;-0.071199692085376298233967418127576820552349090576171875;-0.465386481424449105492868739020195789635181427001953125;-0.65190203212184283376728899384033866226673126220703125;0.196417295595660623686029566670185886323451995849609375;1.328273363123290806697696098126471042633056640625]
  "IW{1,1}(45,:)'" : Constant  Value=[0.08328066219606085340831924668236752040684223175048828125;-0.0086387200980848032061398811265462427400052547454833984375;4.03914922244798990647041136980988085269927978515625;1.739973292628723466890505733317695558071136474609375;1.2728956381039797651766320996102876961231231689453125;1.6218383440950792095947008419898338615894317626953125;-0.272622300615700974280031232410692609846591949462890625;-1.572051328026443428598213358782231807708740234375;1.5634015779536134527205604172195307910442352294921875]
  "IW{1,1}(46,:)'" : Constant  Value=[-0.1785687107336833834292377787278383038938045501708984375;0.38064268559777214573358605775865726172924041748046875;-0.80756423700654444974844636817579157650470733642578125;1.1039065850258122924998360758763737976551055908203125;0.6283498833702498842512795818038284778594970703125;-1.1399469255622409757933155560749582946300506591796875;0.9491270490990781905082940284046344459056854248046875;-0.09058474687432581384793905954211368225514888763427734375;0.09219333781296190633014475679374299943447113037109375]
  "IW{1,1}(47,:)'" : Constant  Value=[0.896138431919418554372214202885515987873077392578125;-0.65539414576085996966270386110409162938594818115234375;-0.99508309562698860073481910148984752595424652099609375;1.80256599312630338971530363778583705425262451171875;2.554112123264038469727665869868360459804534912109375;-4.9327703472042543353381915949285030364990234375;2.180137574288273594191878146375529468059539794921875;1.297765863795575569383800029754638671875;1.301627215941651538599899140535853803157806396484375]
  "IW{1,1}(48,:)'" : Constant  Value=[-0.176506000761501080642545957744005136191844940185546875;1.0501156535890736609673012935672886669635772705078125;-0.36067009568420649312514569828636012971401214599609375;0.4022089913752362466681233854615129530429840087890625;-0.70961864835813182050827663260861299932003021240234375;-0.19649219957758390364688239060342311859130859375;0.91812521554386794520041803480125963687896728515625;-0.5163372709924451964269564996357075870037078857421875;1.1620057726559462896176455615204758942127227783203125]
  "IW{1,1}(49,:)'" : Constant  Value=[1.7933943057759209604995476183830760419368743896484375;2.998418218684526959094682752038352191448211669921875;-0.7974965640670055311289843302802182734012603759765625;0.9453901467701906202734107864671386778354644775390625;-1.688814850904329478709087197785265743732452392578125;-2.085194547328616199166617661830969154834747314453125;-0.51515513431409665212612480900133959949016571044921875;0.7231569230916734536407375344424508512020111083984375;-1.534897526818133517423348166630603373050689697265625]
  "IW{1,1}(5,:)'" : Constant  Value=[0.5499636143825117340355745909619145095348358154296875;0.16347320583180480202400985945132561028003692626953125;0.26825638378688465568444598829955793917179107666015625;-0.373640060294920861583278792750206775963306427001953125;0.295431019089931912180446715865400619804859161376953125;-0.015655106146039786396695348003049730323255062103271484375;-0.491234531054392575821765376531402580440044403076171875;-2.49741940508122706177118743653409183025360107421875;-1.3512683637687465942889275538618676364421844482421875]
  "IW{1,1}(50,:)'" : Constant  Value=[-3.48998432731916619076173446956090629100799560546875;-0.59206397490851048193150063525536097586154937744140625;-0.62064331707214959177321134120575152337551116943359375;0.54068395877625163858937185068498365581035614013671875;3.751236682367735664200836254167370498180389404296875;1.2997700469876132256530354425194673240184783935546875;-2.307138662466164280573366340831853449344635009765625;-0.11239471791295317648629037421414977870881557464599609375;-7.8295908182906988059812647406943142414093017578125]
  "IW{1,1}(6,:)'" : Constant  Value=[-1.3608316413374417219728229611064307391643524169921875;-0.02165616626861564808503857193500152789056301116943359375;-0.2587321613211928106323966858326457440853118896484375;0.52661340109460563763121854208293370902538299560546875;-0.339777447917713193437094787441310472786426544189453125;0.1842263087425662082541322206452605314552783966064453125;0.24697810976838974195146647616638801991939544677734375;-2.92009314945834130838875353219918906688690185546875;2.50867259950981047467166717979125678539276123046875]
  "IW{1,1}(7,:)'" : Constant  Value=[-0.5255948387052347126058293724781833589076995849609375;0.667146172935776604617785778827965259552001953125;-1.0790780012451370861725763461436145007610321044921875;-3.14713128315792456390909137553535401821136474609375;1.4150740412133380186077147300238721072673797607421875;-2.49330509471498107387787968036718666553497314453125;-3.743380325115186479933981900103390216827392578125;0.582432253970156299516247599967755377292633056640625;3.253583275050467182865077120368368923664093017578125]
  "IW{1,1}(8,:)'" : Constant  Value=[2.691557293853317656129320312174968421459197998046875;-3.080997430083618038310078190988861024379730224609375;0.2174028358509282610189217166407615877687931060791015625;0.00779407003777352232198882830971342627890408039093017578125;0.98027367863220760124676189661840908229351043701171875;0.005076694022986778798145479640879784710705280303955078125;-1.3928582263637583338322656345553696155548095703125;0.08157443909133622883533831782187917269766330718994140625;-3.03753286116232512625856543309055268764495849609375]
  "IW{1,1}(9,:)'" : Constant  Value=[0.979717451565743413510745085659436881542205810546875;1.9789958655782788898847002201364375650882720947265625;-3.84912407322519101171565125696361064910888671875;-1.0927005707498953501755067918566055595874786376953125;0.50700311762324634656806665589101612567901611328125;0.25545467502539376258852144019328989088535308837890625;-2.836531331685679280241174637922085821628570556640625;0.6857087236149961295694765794905833899974822998046875;2.25277877930852010734952273196540772914886474609375]
  Mux : Mux  Inputs=50
  dotprod{1..50} (50 alike) : neural/Weight Functions/dotprod
  "iz{1,1}" : Outport
  wires:
  "IW{1,1}(1,:)'"/1 -> dotprod1/1
  "pd{1,1}"/1 -> dotprod1/2, dotprod2/2, dotprod3/2, dotprod4/2, dotprod5/2, dotprod6/2, dotprod7/2, dotprod8/2, dotprod9/2, dotprod10/2, dotprod11/2, dotprod12/2, dotprod13/2, dotprod14/2, dotprod15/2, dotprod16/2, dotprod17/2, dotprod18/2, dotprod19/2, dotprod20/2, dotprod21/2, dotprod22/2, dotprod23/2, dotprod24/2, dotprod25/2, dotprod26/2, dotprod27/2, dotprod28/2, dotprod29/2, dotprod30/2, dotprod31/2, dotprod32/2, dotprod33/2, dotprod34/2, dotprod35/2, dotprod36/2, dotprod37/2, dotprod38/2, dotprod39/2, dotprod40/2, dotprod41/2, dotprod42/2, dotprod43/2, dotprod44/2, dotprod45/2, dotprod46/2, dotprod47/2, dotprod48/2, dotprod49/2, dotprod50/2
  dotprod1/1 -> Mux/1
  "IW{1,1}(2,:)'"/1 -> dotprod2/1
  dotprod2/1 -> Mux/2
  "IW{1,1}(3,:)'"/1 -> dotprod3/1
  dotprod3/1 -> Mux/3
  "IW{1,1}(4,:)'"/1 -> dotprod4/1
  dotprod4/1 -> Mux/4
  "IW{1,1}(5,:)'"/1 -> dotprod5/1
  dotprod5/1 -> Mux/5
  "IW{1,1}(6,:)'"/1 -> dotprod6/1
  dotprod6/1 -> Mux/6
  "IW{1,1}(7,:)'"/1 -> dotprod7/1
  dotprod7/1 -> Mux/7
  "IW{1,1}(8,:)'"/1 -> dotprod8/1
  dotprod8/1 -> Mux/8
  "IW{1,1}(9,:)'"/1 -> dotprod9/1
  dotprod9/1 -> Mux/9
  "IW{1,1}(10,:)'"/1 -> dotprod10/1
  dotprod10/1 -> Mux/10
  "IW{1,1}(11,:)'"/1 -> dotprod11/1
  dotprod11/1 -> Mux/11
  "IW{1,1}(12,:)'"/1 -> dotprod12/1
  dotprod12/1 -> Mux/12
  "IW{1,1}(13,:)'"/1 -> dotprod13/1
  dotprod13/1 -> Mux/13
  "IW{1,1}(14,:)'"/1 -> dotprod14/1
  dotprod14/1 -> Mux/14
  "IW{1,1}(15,:)'"/1 -> dotprod15/1
  dotprod15/1 -> Mux/15
  "IW{1,1}(16,:)'"/1 -> dotprod16/1
  dotprod16/1 -> Mux/16
  "IW{1,1}(17,:)'"/1 -> dotprod17/1
  dotprod17/1 -> Mux/17
  "IW{1,1}(18,:)'"/1 -> dotprod18/1
  dotprod18/1 -> Mux/18
  "IW{1,1}(19,:)'"/1 -> dotprod19/1
  dotprod19/1 -> Mux/19
  "IW{1,1}(20,:)'"/1 -> dotprod20/1
  dotprod20/1 -> Mux/20
  "IW{1,1}(21,:)'"/1 -> dotprod21/1
  dotprod21/1 -> Mux/21
  "IW{1,1}(22,:)'"/1 -> dotprod22/1
  dotprod22/1 -> Mux/22
  "IW{1,1}(23,:)'"/1 -> dotprod23/1
  dotprod23/1 -> Mux/23
  "IW{1,1}(24,:)'"/1 -> dotprod24/1
  dotprod24/1 -> Mux/24
  "IW{1,1}(25,:)'"/1 -> dotprod25/1
  dotprod25/1 -> Mux/25
  "IW{1,1}(26,:)'"/1 -> dotprod26/1
  dotprod26/1 -> Mux/26
  "IW{1,1}(27,:)'"/1 -> dotprod27/1
  dotprod27/1 -> Mux/27
  "IW{1,1}(28,:)'"/1 -> dotprod28/1
  dotprod28/1 -> Mux/28
  "IW{1,1}(29,:)'"/1 -> dotprod29/1
  dotprod29/1 -> Mux/29
  "IW{1,1}(30,:)'"/1 -> dotprod30/1
  dotprod30/1 -> Mux/30
  "IW{1,1}(31,:)'"/1 -> dotprod31/1
  dotprod31/1 -> Mux/31
  "IW{1,1}(32,:)'"/1 -> dotprod32/1
  dotprod32/1 -> Mux/32
  "IW{1,1}(33,:)'"/1 -> dotprod33/1
  dotprod33/1 -> Mux/33
  "IW{1,1}(34,:)'"/1 -> dotprod34/1
  dotprod34/1 -> Mux/34
  "IW{1,1}(35,:)'"/1 -> dotprod35/1
  dotprod35/1 -> Mux/35
  "IW{1,1}(36,:)'"/1 -> dotprod36/1
  dotprod36/1 -> Mux/36
  "IW{1,1}(37,:)'"/1 -> dotprod37/1
  dotprod37/1 -> Mux/37
  "IW{1,1}(38,:)'"/1 -> dotprod38/1
  dotprod38/1 -> Mux/38
  "IW{1,1}(39,:)'"/1 -> dotprod39/1
  dotprod39/1 -> Mux/39
  "IW{1,1}(40,:)'"/1 -> dotprod40/1
  dotprod40/1 -> Mux/40
  "IW{1,1}(41,:)'"/1 -> dotprod41/1
  dotprod41/1 -> Mux/41
  "IW{1,1}(42,:)'"/1 -> dotprod42/1
  dotprod42/1 -> Mux/42
  "IW{1,1}(43,:)'"/1 -> dotprod43/1
  dotprod43/1 -> Mux/43
  "IW{1,1}(44,:)'"/1 -> dotprod44/1
  dotprod44/1 -> Mux/44
  "IW{1,1}(45,:)'"/1 -> dotprod45/1
  dotprod45/1 -> Mux/45
  "IW{1,1}(46,:)'"/1 -> dotprod46/1
  dotprod46/1 -> Mux/46
  "IW{1,1}(47,:)'"/1 -> dotprod47/1
  dotprod47/1 -> Mux/47
  "IW{1,1}(48,:)'"/1 -> dotprod48/1
  dotprod48/1 -> Mux/48
  "IW{1,1}(49,:)'"/1 -> dotprod49/1
  dotprod49/1 -> Mux/49
  "IW{1,1}(50,:)'"/1 -> dotprod50/1
  dotprod50/1 -> Mux/50
  Mux/1 -> "iz{1,1}"/1

== system nnROSNode/Neural Network/Function Fitting Neural Network1/Layer 2/Delays 1 ==
  "p{2}" : Inport  PortDimensions=50
  mux : Mux  Inputs=1
  "pd{2,1}" : Outport
  wires:
  "p{2}"/1 -> mux/1
  mux/1 -> "pd{2,1}"/1
